simulink model "Allegato1"  (R2022b)
settings: Solver=VariableStepAuto  StartTime=0.0  StopTime=40  RelTol=1e-3
libraries: SignalEditorBlockLib x1
settings Model: Creator=andre  LastModifiedBy=andre

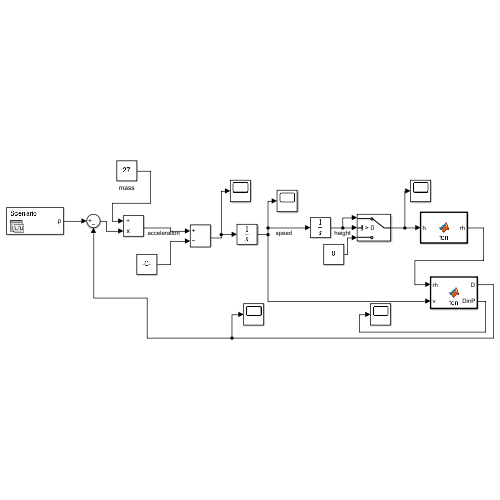
[thumbnail: Simulink's stored preview of the top-level diagram]
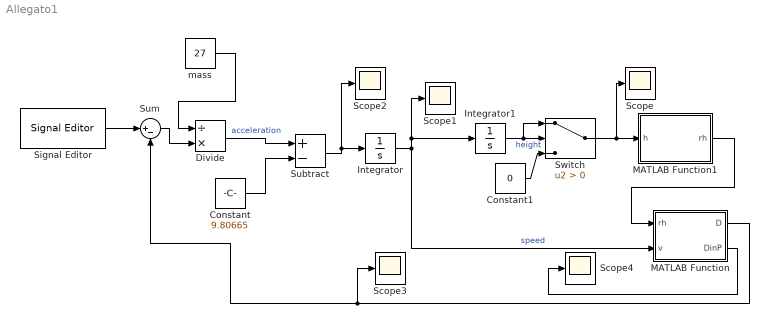
== system Allegato1 ==
  Constant : Constant  Value=9.80665
  Constant1 : Constant  Value=0
  Divide : Product  Inputs=/*
  Integrator : Integrator
  Integrator1 : Integrator
  MATLAB Function : MATLAB Function  TreatAsAtomicUnit=on
  MATLAB Function1 : MATLAB Function  TreatAsAtomicUnit=on
  Scope{,1..4} (5 alike) : Scope
  Signal Editor : SignalEditorBlockLib/Signal Editor  FileName=C:\Users\andre\Desktop\ANDREA_STEFANI\Allegati\AeroTech_M2000R.mat  ActiveScenario=Scenario  ActiveSignal=p  IsBus=off  OutputBusObjectStr=Bus: BusObject  SampleTime=0  Interpolate=off  ZeroCross=off  OutputAfterFinalValue=Setting to zero  Unit=inherit  PreserveSignalName=on
  Subtract : Sum  Inputs=+-
  Sum : Sum  Inputs=|+-
  Switch : Switch  Criteria=u2 > Threshold  SaturateOnIntegerOverflow=off  InputSameDT=off
  mass : Constant  Value=27
  wires:
  mass/1 -> Divide/1
  Integrator/1 -> Scope1/1, Integrator1/1, MATLAB Function/2(v)  "speed"
  Divide/1 -> Subtract/1  "acceleration"
  Subtract/1 -> Scope2/1, Integrator/1
  Constant/1 -> Subtract/2
  MATLAB Function/1(D) -> Sum/2, Scope3/1
  Switch/1 -> Scope/1, MATLAB Function1/1(h)
  Integrator1/1 -> Switch/1, Switch/2  "height"
  Constant1/1 -> Switch/3
  MATLAB Function1/1(rh) -> MATLAB Function/1(rh)
  MATLAB Function/2(DinP) -> Scope4/1
  Signal Editor/1 -> Sum/1
  Sum/1 -> Divide/2

== matlab function Allegato1/MATLAB Function ==
  data: rh input; D output; v input; DinP output
function [D, DinP]= fcn(rh, v)
cd=0.36;
S=pi*0.075^2;
DinP=0.5*rh*v^2;
D = DinP*S*cd;

== matlab function Allegato1/MATLAB Function1 ==
  data: h input; rh output
function rh = fcn(h)
rh0=1.2250
g0=9.80665
M=0.0289644 %molar mass of air
R=8.3144598
T=288.15
rh = rh0*exp(-g0*M*h/(R*T));
